simulink model "pvsimulation"  (R2014b)
settings: Solver=ode45  StartTime=0.0  StopTime=10  MaxStep=0.01  MinStep=0.01  RelTol=1e-3
undefined symbols (not defined in the file or in its folder): sigbuilder_block
libraries: simulink x3
settings Model: CovSFcnEnable=on  Creator=TCM  LastModifiedBy=root
settings OptimizationCC: UseDivisionForNetSlopeComputation=off  SimCompilerOptimization=off
settings DebuggingCC: UnderspecifiedInitializationDetection=Classic  MergeDetectMultiDrivingBlocksExec=none  FrameProcessingCompatibilityMsg=error  StateNameClashWarn=warning
settings RTWCC: RTWCompilerOptimization=off

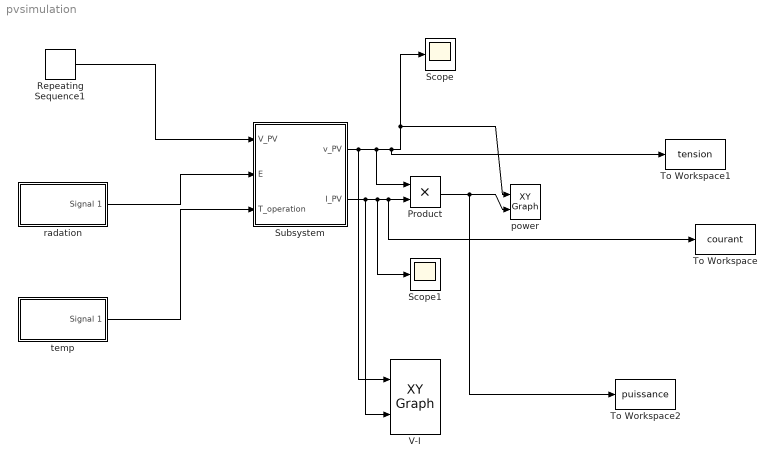
== system pvsimulation ==
  Product : Product
  Repeating Sequence1 : simulink/Sources/Repeating Sequence  rep_seq_t=[0 1 2]  rep_seq_y=[0 40 0 ]
  Scope : Scope
  Scope1 : Scope
  Subsystem : Subsystem
  To Workspace : ToWorkspace  VariableName=courant  SampleTime=-1
  To Workspace1 : ToWorkspace  VariableName=tension  SampleTime=-1
  To Workspace2 : ToWorkspace  VariableName=puissance  SampleTime=-1
  "V-I " : simulink/Sinks/XY Graph  xmin=0  xmax=37  ymin=0  ymax=12  st=-1
  power : simulink/Sinks/XY Graph  xmin=0  xmax=37  ymin=0  ymax=400  st=-1
  radation : Subsystem  Tag=STV Subsys  LoadFcn=sigbuilder_block('load');  StartFcn=sigbuilder_block('start');  StopFcn=sigbuilder_block('stop');  ClipboardFcn=sigbuilder_block('clipboard');  mask(Sigbuilder block){}
      mask help: Simulink:masks:SigbuilderBlock_MD
      mask init:
      | if ~strcmp(get_param(bdroot(gcbh),'SimulationStatus'),'stopped') tuvar = sigbuilder_block('maskInit'); end
      settings: CopyFcn=sigbuilder_block('copy');  DeleteFcn=sigbuilder_block('delete');  ModelCloseFcn=sigbuilder_block('modelClose');  PreSaveFcn=sigbuilder_block('preSave');  PauseFcn=sigbuilder_block('pause');  ContinueFcn=sigbuilder_block('continue');  NameChangeFcn=sigbuilder_block('namechange');  OpenFcn=sigbuilder_block('open',[267 58.5 550.5 394.5 ]);  CloseFcn=sigbuilder_block('close');
      mask Display: plot(0, 0, 100, 100,[2, 2, 32, 32, 2], [68, 8, 8, 68, 68],[32, 2], [38, 38], [32, 19, 2],[53, 60, 44], [32, 17, 17, 2],[16, 16, 31, 31]);txt = getActiveGroup(gcbh);text(2, 100, txt,'verticalAlignment', 'top');
  temp : Subsystem  Tag=STV Subsys  LoadFcn=sigbuilder_block('load');  StartFcn=sigbuilder_block('start');  StopFcn=sigbuilder_block('stop');  ClipboardFcn=sigbuilder_block('clipboard');  mask(Sigbuilder block){}
      mask help: Simulink:masks:SigbuilderBlock_MD
      mask init:
      | if ~strcmp(get_param(bdroot(gcbh),'SimulationStatus'),'stopped') tuvar = sigbuilder_block('maskInit'); end
      settings: CopyFcn=sigbuilder_block('copy');  DeleteFcn=sigbuilder_block('delete');  ModelCloseFcn=sigbuilder_block('modelClose');  PreSaveFcn=sigbuilder_block('preSave');  PauseFcn=sigbuilder_block('pause');  ContinueFcn=sigbuilder_block('continue');  NameChangeFcn=sigbuilder_block('namechange');  OpenFcn=sigbuilder_block('open',[437.25 118.5 550.5 394.5 ]);  CloseFcn=sigbuilder_block('close');
      mask Display: plot(0, 0, 100, 100,[2, 2, 32, 32, 2], [68, 8, 8, 68, 68],[32, 2], [38, 38], [32, 19, 2],[53, 60, 44], [32, 17, 17, 2],[16, 16, 31, 31]);txt = getActiveGroup(gcbh);text(2, 100, txt,'verticalAlignment', 'top');
  wires:
  Subsystem/1(v_PV) -> "V-I "/1, Product/1, To Workspace1/1, power/1, Scope/1
  Subsystem/2(I_PV) -> "V-I "/2, Scope1/1, To Workspace/1, Product/2
  Repeating Sequence1/1 -> Subsystem/1(V_PV)
  Product/1 -> To Workspace2/1, power/2
  radation/1(Signal 1) -> Subsystem/2(E)
  temp/1(Signal 1) -> Subsystem/3(T_operation)

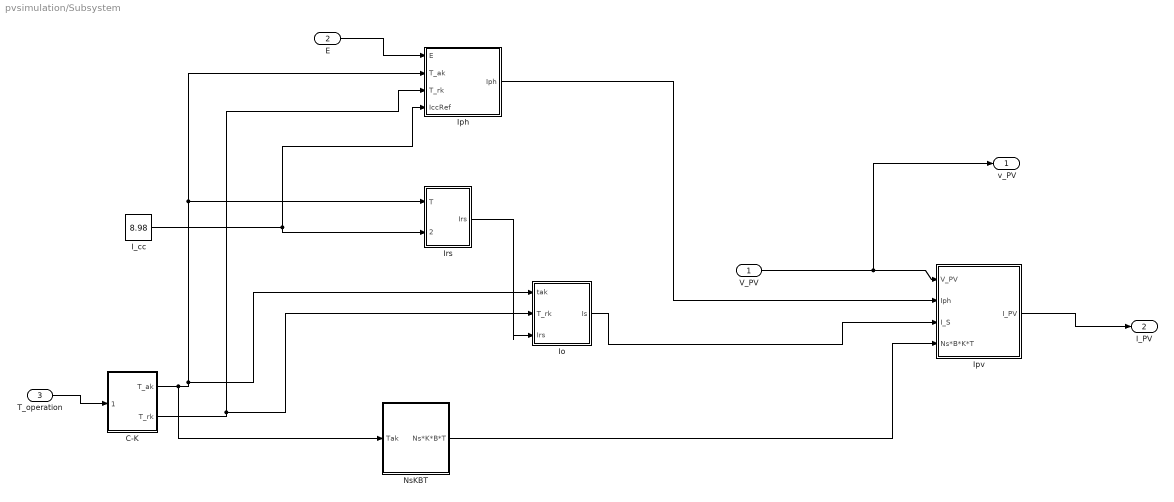
== system pvsimulation/Subsystem ==
  V_PV : Inport
  E : Inport  Port=2
  T_operation : Inport  Port=3
  C-K : Subsystem
  I_cc : Constant  Value=8.98
  Io : Subsystem
  Iph : Subsystem
  Ipv : Subsystem
  Irs : Subsystem
  NsKBT : Subsystem
  v_PV : Outport
  I_PV : Outport  Port=2
  wires:
  T_operation/1 -> C-K/1(T_operation)
  E/1 -> Iph/1(E)
  C-K/2(T_rk) -> Iph/3(T_rk), Io/2(T_rk)
  I_cc/1 -> Iph/4(IccRef), Irs/2(Icc_ref)
  NsKBT/1(Ns*K*B*T) -> Ipv/4(Ns*B*K*T)
  Irs/1(Irs) -> Io/3(Irs)
  C-K/1(T_ak) -> NsKBT/1(Tak), Irs/1(T), Iph/2(T_ak), Io/1(tak)
  Iph/1(Iph) -> Ipv/2(Iph)
  Ipv/1(I_PV) -> I_PV/1
  Io/1(Is) -> Ipv/3(I_S)
  V_PV/1 -> v_PV/1, Ipv/1(V_PV)

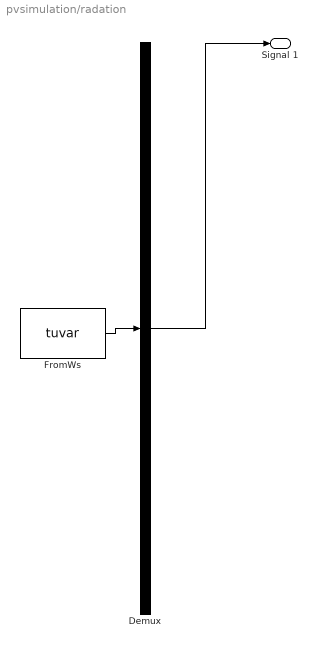
== system pvsimulation/radation ==
  Demux : Demux  Tag=STV Demux  Outputs=1
  FromWs : FromWorkspace  Tag=STV FromWs  VariableName=tuvar  SampleTime=0
      SigBuilderData=|
      | common.afterFinalStr = 'Extrapolate'
      | common.sampleTime = 0
      | dataSet.timeRange = [0 10]
      | dataSet.name = 'Group 1'
      | sbobj.Groups.Name = 'Group 1'
      | sbobj.Groups.Signals.Name = 'Signal 1'
      | sbobj.Groups.Signals.XData = [0 1 2 10]
      | sbobj.Groups.Signals.YData = [1000 1000 1000 1000]
  Signal 1 : Outport  Tag=STV Outport
  wires:
  FromWs/1 -> Demux/1
  Demux/1 -> Signal 1/1

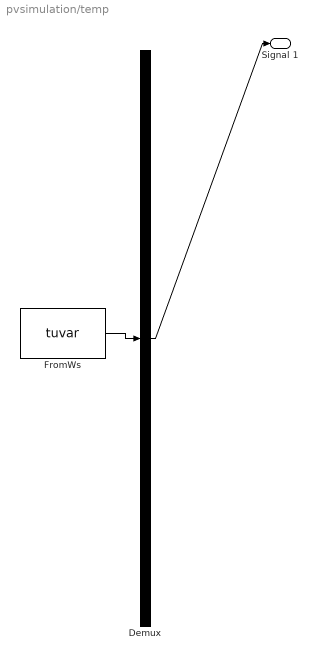
== system pvsimulation/temp ==
  Demux : Demux  Tag=STV Demux  Outputs=1
  FromWs : FromWorkspace  Tag=STV FromWs  VariableName=tuvar  SampleTime=0
      SigBuilderData=|
      | common.afterFinalStr = 'Extrapolate'
      | common.sampleTime = 0
      | dataSet.timeRange = [0 10]
      | dataSet.name = 'Group 1'
      | sbobj.Groups.Name = 'Group 1'
      | sbobj.Groups.Signals.Name = 'Signal 1'
      | sbobj.Groups.Signals.XData = [0 4 6 10]
      | sbobj.Groups.Signals.YData = [25 25 25 25]
  Signal 1 : Outport  Tag=STV Outport
  wires:
  FromWs/1 -> Demux/1
  Demux/1 -> Signal 1/1

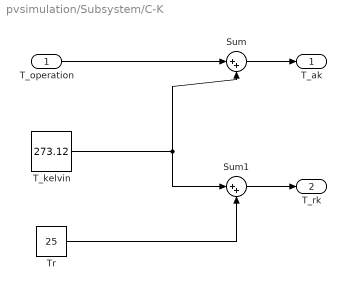
== system pvsimulation/Subsystem/C-K ==
  T_operation : Inport
  Sum : Sum  Inputs=|++
  Sum1 : Sum  Inputs=|++
  T_kelvin : Constant  Value=273.12
  Tr : Constant  Value=25
  T_ak : Outport
  T_rk : Outport  Port=2
  wires:
  T_kelvin/1 -> Sum1/1, Sum/2
  T_operation/1 -> Sum/1
  Tr/1 -> Sum1/2
  Sum/1 -> T_ak/1
  Sum1/1 -> T_rk/1

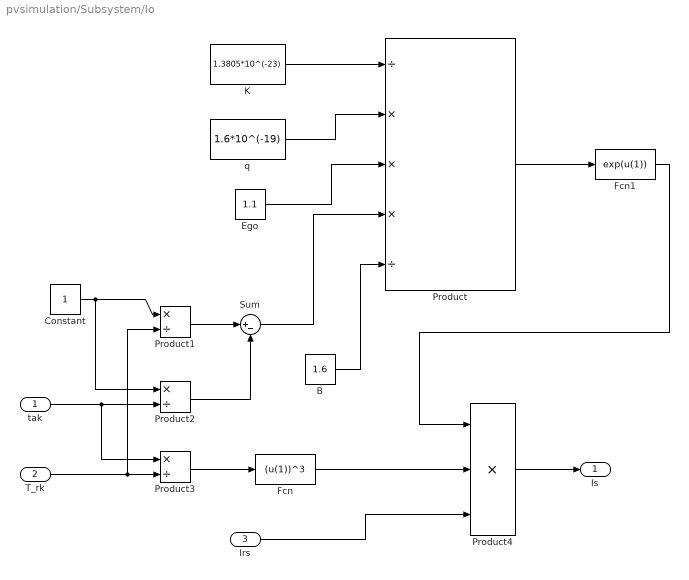
== system pvsimulation/Subsystem/Io ==
  tak : Inport
  T_rk : Inport  Port=2
  Irs : Inport  Port=3
  B : Constant  Value=1.6
  Constant : Constant
  Ego : Constant  Value=1.1
  Fcn : Fcn  Expr=(u(1))^3
  Fcn1 : Fcn  Expr=exp(u(1))
  K : Constant  Value=1.3805*10^(-23)
  Product : Product  Inputs=/***/
  Product1 : Product  Inputs=*/
  Product2 : Product  Inputs=*/
  Product3 : Product  Inputs=*/
  Product4 : Product  Inputs=3
  Sum : Sum  Inputs=|+-
  q : Constant  Value=1.6*10^(-19)
  Is : Outport
  wires:
  q/1 -> Product/2
  K/1 -> Product/1
  Product2/1 -> Sum/2
  Irs/1 -> Product4/3
  Ego/1 -> Product/3
  Sum/1 -> Product/4
  Product3/1 -> Fcn/1
  Product1/1 -> Sum/1
  Constant/1 -> Product2/1, Product1/1
  B/1 -> Product/5
  tak/1 -> Product3/1, Product2/2
  Fcn/1 -> Product4/2
  Product/1 -> Fcn1/1
  Fcn1/1 -> Product4/1
  T_rk/1 -> Product1/2, Product3/2
  Product4/1 -> Is/1

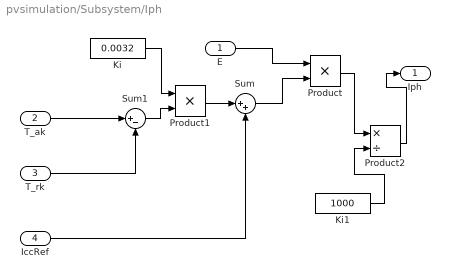
== system pvsimulation/Subsystem/Iph ==
  E : Inport
  T_ak : Inport  Port=2
  T_rk : Inport  Port=3
  IccRef : Inport  Port=4
  Ki : Constant  Value=0.0032
  Ki1 : Constant  Value=1000
  Product : Product
  Product1 : Product
  Product2 : Product  Inputs=*/
  Sum : Sum  Inputs=|++
  Sum1 : Sum  Inputs=|+-
  Iph : Outport
  wires:
  E/1 -> Product/1
  T_ak/1 -> Sum1/1
  T_rk/1 -> Sum1/2
  Sum/1 -> Product/2
  IccRef/1 -> Sum/2
  Product1/1 -> Sum/1
  Ki/1 -> Product1/1
  Sum1/1 -> Product1/2
  Product/1 -> Product2/1
  Ki1/1 -> Product2/2
  Product2/1 -> Iph/1

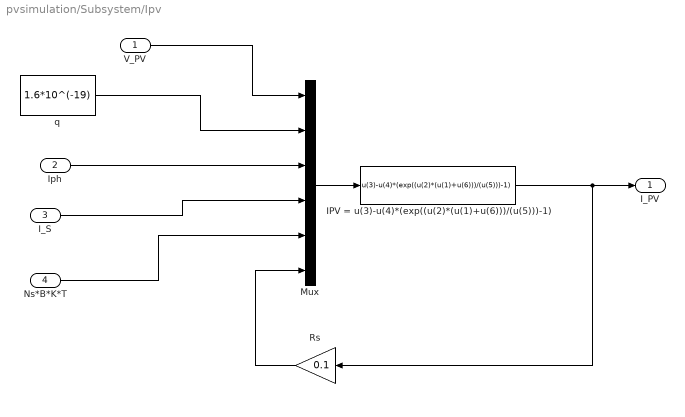
== system pvsimulation/Subsystem/Ipv ==
  V_PV : Inport
  Iph : Inport  Port=2
  I_S : Inport  Port=3
  Ns*B*K*T : Inport  Port=4
  IPV = u(3)-u(4)*(exp((u(2)*(u(1)+u(6)))/(u(5)))-1) : Fcn  Expr=u(3)-u(4)*(exp((u(2)*(u(1)+u(6)))/(u(5)))-1)
  Mux : Mux  Inputs=6
  Rs : Gain  Gain=0.1
  q : Constant  Value=1.6*10^(-19)
  I_PV : Outport
  wires:
  IPV = u(3)-u(4)*(exp((u(2)*(u(1)+u(6)))/(u(5)))-1)/1 -> I_PV/1, Rs/1
  Ns*B*K*T/1 -> Mux/5
  Mux/1 -> IPV = u(3)-u(4)*(exp((u(2)*(u(1)+u(6)))/(u(5)))-1)/1
  I_S/1 -> Mux/4
  Rs/1 -> Mux/6
  q/1 -> Mux/2
  Iph/1 -> Mux/3
  V_PV/1 -> Mux/1

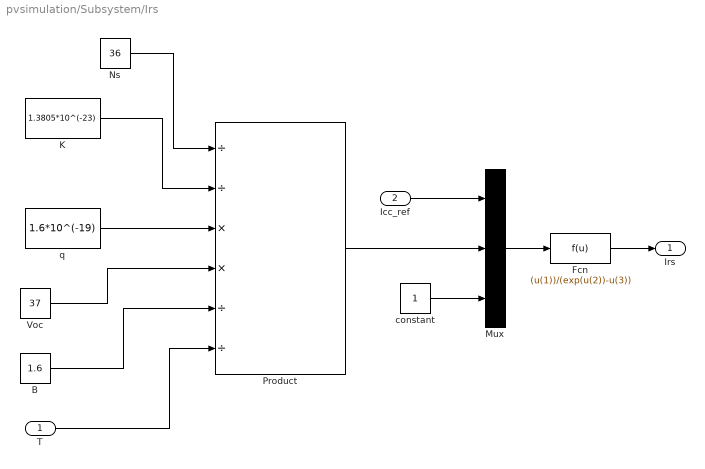
== system pvsimulation/Subsystem/Irs ==
  T : Inport
  Icc_ref : Inport  Port=2
  B : Constant  Value=1.6
  Fcn : Fcn  Expr=(u(1))/(exp(u(2))-u(3))
  K : Constant  Value=1.3805*10^(-23)
  Mux : Mux  Inputs=3
  Ns : Constant  Value=36
  Product : Product  Inputs=//**//
  Voc : Constant  Value=37
  constant : Constant
  q : Constant  Value=1.6*10^(-19)
  Irs : Outport
  wires:
  Ns/1 -> Product/1
  K/1 -> Product/2
  q/1 -> Product/3
  B/1 -> Product/5
  Voc/1 -> Product/4
  T/1 -> Product/6
  Product/1 -> Mux/2
  Icc_ref/1 -> Mux/1
  constant/1 -> Mux/3
  Mux/1 -> Fcn/1
  Fcn/1 -> Irs/1

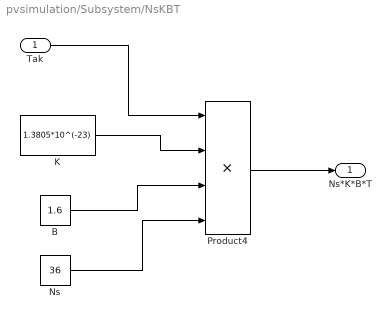
== system pvsimulation/Subsystem/NsKBT ==
  Tak : Inport
  B : Constant  Value=1.6
  K : Constant  Value=1.3805*10^(-23)
  Ns : Constant  Value=36
  Product4 : Product  Inputs=4
  Ns*K*B*T : Outport
  wires:
  Product4/1 -> Ns*K*B*T/1
  K/1 -> Product4/2
  B/1 -> Product4/3
  Tak/1 -> Product4/1
  Ns/1 -> Product4/4
